simulink model "drive_around"  (R2017b)
settings: Solver=FixedStepAuto  StartTime=0.0  StopTime=inf  FixedStep=0.05  RelTol=1e-3
undefined symbols (not defined in the file or in its folder): Angular, Linear
libraries: robotlib x3, aerolibanimutils x1
settings Model: Creator=scastro  LastModifiedBy=scastro
settings OptimizationCC: PassReuseOutputArgsAs=Individual arguments  MaxStackSize=64
settings DebuggingCC: ParameterTunabilityLossMsg=error
settings HardwareCC: ProdBitPerPointer=32  ProdBitPerSizeT=32  ProdBitPerPtrDiffT=32  ProdLargestAtomicFloat=None  ProdIntDivRoundTo=Undefined  ProdEndianess=Unspecified  ProdWordSize=32  ProdHWDeviceType=Generic->Unspecified (assume 32-bit Generic)
settings SFSimCC: MATLABDynamicMemAlloc=off
settings RTWCC: SystemTargetFile=ert.tlc  HardwareBoard=Robot Operating System (ROS)  TemplateMakefile=ert_default_tmf  GenerateReport=on  Toolchain=Catkin  IncludeHyperlinkInReport=on  LaunchReport=on  TargetLang=C++  GenerateTraceInfo=on  GenerateTraceReport=on  GenerateTraceReportSl=on  GenerateTraceReportSf=on  GenerateTraceReportEml=on
settings CodeAppCC: ForceParamTrailComments=on  IgnoreCustomStorageClasses=off  OperatorAnnotations=on  SimulinkDataObjDesc=on  SFDataObjDesc=on  InsertBlockDesc=on

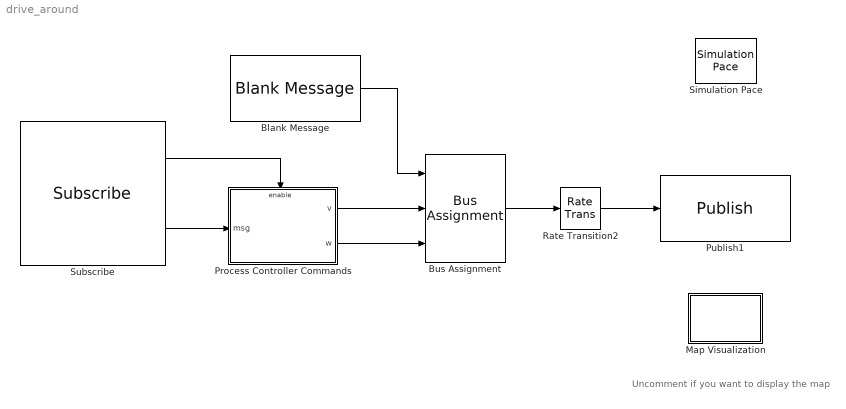
== system drive_around ==
  note: Uncomment if you want to display the map
  Blank Message : robotlib/Blank Message  SourceLibraryInfo=This block requires Robotics System Toolbox  messageType=geometry_msgs/Twist  SampleTime=inf
      settings: SourceProductBaseCode=RO
  Bus Assignment : BusAssignment  DialogController=Simulink.DDGSource_BusAssignment  AssignedSignals=Linear.X,Angular.Z
  Map Visualization : MATLAB Function  TreatAsAtomicUnit=on  mask(Map Visualization){plotUpdateTime=5}
      mask prompts: plotUpdateTime "Plot update time:"
      mask help: Subscribes to the /map ROS topic and displays the latest occupancy grid received over the network.
  Process Controller Commands : Subsystem  TreatAsAtomicUnit=on
  Publish1 : robotlib/Publish  SourceLibraryInfo=This block requires Robotics System Toolbox  topicSource=Select from ROS network  topic=/mobile_base/commands/velocity  messageType=geometry_msgs/Twist  messageQueueLength=105
      settings: SourceProductBaseCode=RO
  Rate Transition2 : RateTransition
  Simulation Pace : aerolibanimutils/Simulation Pace  SimulationPace=1  SleepMode=MATLAB Thread  OutputPaceError=off  SampleTime=0.05
  Subscribe : robotlib/Subscribe  SourceLibraryInfo=This block requires Robotics System Toolbox  topicSource=Select from ROS network  topic=/joy  messageType=sensor_msgs/Joy  sampleTime=-1  messageQueueLength=1
      settings: SourceProductBaseCode=RO
  wires:
  Subscribe/1 -> Process Controller Commands/Enable
  Subscribe/2 -> Process Controller Commands/1(msg)
  Rate Transition2/1 -> Publish1/1
  Process Controller Commands/2(w) -> Bus Assignment/3
  Process Controller Commands/1(v) -> Bus Assignment/2
  Bus Assignment/1 -> Rate Transition2/1
  Blank Message/1 -> Bus Assignment/1

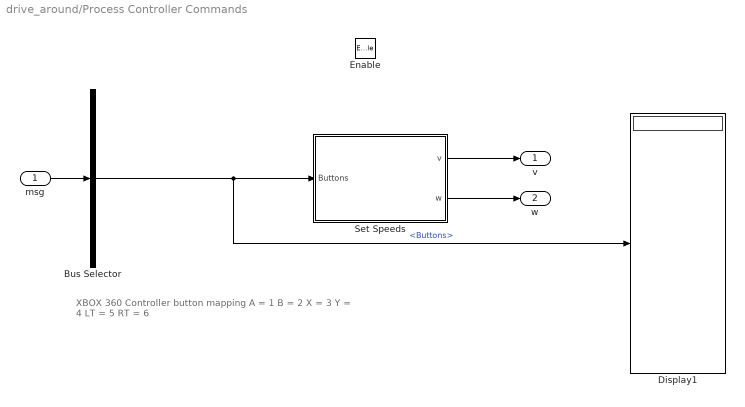
== system drive_around/Process Controller Commands ==
  note: XBOX 360 Controller button mapping
      | A = 1
      | B = 2
      | X = 3
      | Y = 4
      | LT = 5
      | RT = 6
  msg : Inport
  Enable : EnablePort  StatesWhenEnabling=reset
  Bus Selector : BusSelector  OutputSignals=Buttons
  Display1 : Display
  Set Speeds : Stateflow chart  TreatAsAtomicUnit=on
  v : Outport
  w : Outport  Port=2
  wires:
  msg/1 -> Bus Selector/1
  Bus Selector/1 -> Display1/1, Set Speeds/1(Buttons)  "<Buttons>"
  Set Speeds/1(v) -> v/1
  Set Speeds/2(w) -> w/1

== matlab function drive_around/Map Visualization ==
  settings: updateMethod=DISCRETE  sampleTime=plotUpdateTime
function visualizeMap

    coder.extrinsic('showMap');
    showMap;
    
end

== stateflow chart drive_around/Process Controller Commands/Set Speeds ==
  (default) -> (junction 25) : {
      | A = Buttons(1);
      | B = Buttons(2);
      | X = Buttons(3);
      | Y = Buttons(4);
      | RT = Buttons(6);
      | }
  (junction 25) -> (junction 26) [order 1] : [Y]
  (junction 25) -> (junction 27) [order 2]
  (junction 26) -> (junction 31) : {v = 0.2;}
  (junction 27) -> (junction 28) [order 1] : [A]
  (junction 27) -> (junction 29) [order 2] : {v = 0;}
  (junction 28) -> (junction 30) : {v = -0.2;}
  (junction 30) -> (junction 29)
  (junction 31) -> (junction 30)
  (junction 29) -> (junction 45)
  (junction 45) -> (junction 46) [order 1] : [X]
  (junction 45) -> (junction 47) [order 2]
  (junction 46) -> (junction 41) : {w = 0.75;}
  (junction 47) -> (junction 44) [order 1] : [B]
  (junction 47) -> (junction 48) [order 2] : {w = 0;}
  (junction 44) -> (junction 34) : {w = -0.75;}
  (junction 34) -> (junction 48)
  (junction 41) -> (junction 34)
  (junction 48) -> (junction 60)
  (junction 60) -> (junction 61) [order 1] : [RT]
  (junction 60) -> (junction 62) [order 2]
  (junction 61) -> (junction 63) : {v = v*2;}
  (junction 63) -> (junction 62)
  (junction 62) -> (junction 64)
  data: v output; Buttons input; w output; A local; X local; Y local; B local; RT local
